simulink model "Example_for_the_implementation_of_the_inverse_kinematics"  (R2022a)
settings: Solver=FixedStepAuto  StartTime=0.0  StopTime=2  FixedStep=0.01  RelTol=1e-3  EnableMultiTasking=on
InitFcn:
  | %Simu_init
StopFcn:
  | %stop_sim
undefined symbols (not defined in the file): STIFF_FLOP_TipInverse
libraries: arduinolib x12, simulink x2, sldrtlib x1
settings Model: SimulationMode=external  PacingRate=1000  ExtModeTrigDuration=2  Creator=11010  LastModifiedBy=11010
settings SolverCC: AlgebraicLoopSolver=TrustRegion
settings OptimizationCC: EnhancedBackFolding=on  PassReuseOutputArgsAs=Individual arguments  MaxStackSize=64  OptimizeBlockOrder=speed  DifferentSizesBufferReuse=on  OptimizationCustomize=off  EfficientTunableParamExpr=on
settings DebuggingCC: ParameterTunabilityLossMsg=error  UnconnectedInputMsg=warning  UnconnectedOutputMsg=warning  UnconnectedLineMsg=warning  SFMachineParentedDataDiag=warning
settings HardwareCC: ProdBitPerPointer=32  ProdBitPerSizeT=32  ProdBitPerPtrDiffT=32  ProdLargestAtomicInteger=Long  ProdLargestAtomicFloat=Double  ProdWordSize=32  ProdHWDeviceType=ARM Compatible->ARM Cortex
settings SFSimCC: MATLABDynamicMemAlloc=off  CustomCodeUndefinedFunction=UseInterfaceOnly
settings RTWCC: SystemTargetFile=ert.tlc  HardwareBoard=Arduino Due  TemplateMakefile=ert_default_tmf  GenerateReport=on  Toolchain=Arduino ARM  BuildConfiguration=Faster Runs  IncludeHyperlinkInReport=on  LaunchReport=on  GenerateTraceInfo=on  GenerateTraceReport=on  GenerateTraceReportSl=on  GenerateTraceReportSf=on  GenerateTraceReportEml=on
settings CodeAppCC: ForceParamTrailComments=on  IgnoreCustomStorageClasses=off  OperatorAnnotations=on  SimulinkDataObjDesc=on  SFDataObjDesc=on  InsertBlockDesc=on
settings ERTTargetCC: SupportContinuousTime=on  SupportVariableSizeSignals=on  ExtModeTransport=3  ExtModeStaticAlloc=on  ExtModeStaticAllocSize=24576  ExtModeMexFile=ext_xcp  ExtModeIntrfLevel=Level2 - Open

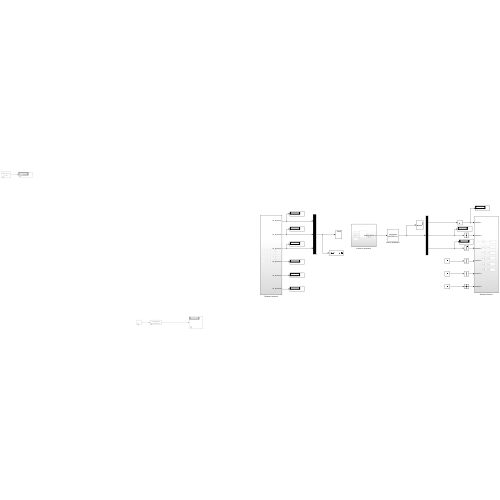
[thumbnail: Simulink's stored preview of the top-level diagram]
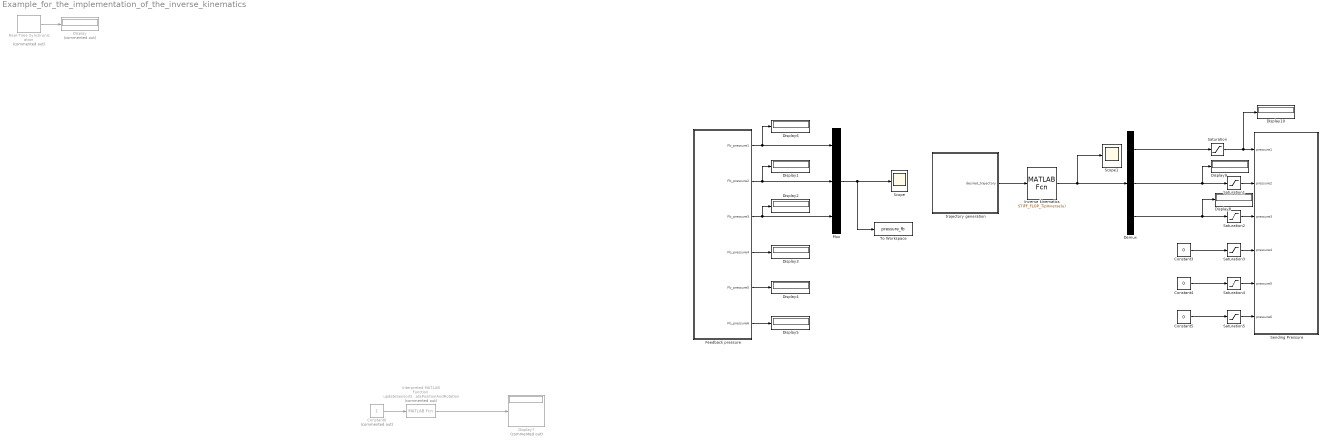
== system Example_for_the_implementation_of_the_inverse_kinematics ==
  Constant3 : Constant  Value=0
  Constant4 : Constant  Value=0
  Constant5 : Constant  Value=0
  Constant6 : Constant  Commented=on
  Demux : Demux  Outputs=3
  Display : Display  Commented=on
  Display{1..6,8..10} (9 alike) : Display
  Display7 : Display  Commented=on
  Feedback pressure : Subsystem
  Interpreted MATLAB Function : MATLABFcn  Commented=on  MATLABFcn=updateSensorDataPositionAndRotation  OutputDimensions=3
  Inverse kinematics : MATLABFcn  MATLABFcn=STIFF_FLOP_TipInverse(u)  OutputDimensions=3
  Mux : Mux  Inputs=3
  Real-Time Synchronization : sldrtlib/Real-Time Synchronization  Commented=on  SampleTime=0.1  MaxMissedTicks=100  ShowMissedTicks=on  YieldWhenWaiting=off
  Saturation{,1..5} (6 alike) : Saturate  UpperLimit=1.5  LowerLimit=0
  Scope : Scope
  Scope1 : Scope
  Sending Pressure : Subsystem
  To Workspace : ToWorkspace  VariableName=pressure_fb  SaveFormat=Structure With Time  SampleTime=-1
  trajectory generation : Subsystem
  wires:
  Demux/3 -> Saturation2/1, Display8/1
  Constant4/1 -> Saturation4/1
  Constant5/1 -> Saturation5/1
  Feedback pressure/2(Fb_pressure2) -> Display1/1, Mux/2
  Feedback pressure/3(Fb_pressure3) -> Display2/1, Mux/3
  Feedback pressure/4(Fb_pressure4) -> Display3/1
  Feedback pressure/5(Fb_pressure5) -> Display4/1
  Feedback pressure/6(Fb_pressure6) -> Display5/1
  Feedback pressure/1(Fb_pressure1) -> Display6/1, Mux/1
  Real-Time Synchronization/1 -> Display/1
  Constant3/1 -> Saturation3/1
  Interpreted MATLAB Function/1 -> Display7/1
  Constant6/1 -> Interpreted MATLAB Function/1
  Saturation/1 -> Display10/1, Sending Pressure/1(pressure1)
  Saturation1/1 -> Sending Pressure/2(pressure2)
  Saturation2/1 -> Sending Pressure/3(pressure3)
  Saturation3/1 -> Sending Pressure/4(pressure4)
  Saturation4/1 -> Sending Pressure/5(pressure5)
  Saturation5/1 -> Sending Pressure/6(pressure6)
  Inverse kinematics/1 -> Scope1/1, Demux/1
  trajectory generation/1(desired_trajectory) -> Inverse kinematics/1
  Mux/1 -> To Workspace/1, Scope/1
  Demux/1 -> Saturation/1
  Demux/2 -> Display9/1, Saturation1/1

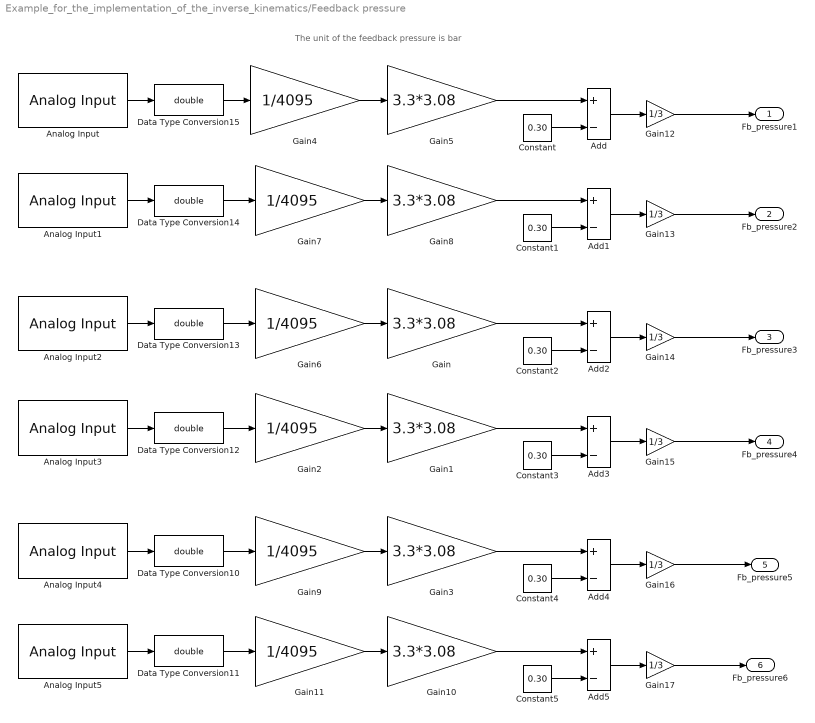
== system Example_for_the_implementation_of_the_inverse_kinematics/Feedback pressure ==
  note: The unit of the feedback pressure is bar
  Add{,1..5} (6 alike) : Sum  Inputs=+-
  Analog Input : arduinolib/Analog Input  pinNumber=0  ReadResultsOnly=off  ConversionTriggerSource=Software  ExternalTriggerType=uint32(0)  OutputDataType=uint16  EnableConversionCompleteNotify=off  EnableOuputStatus=off  SampleTime=0.01  blockPlatform=arduino
  Analog Input1 : arduinolib/Analog Input  pinNumber=1  ReadResultsOnly=off  ConversionTriggerSource=Software  ExternalTriggerType=uint32(0)  OutputDataType=uint16  EnableConversionCompleteNotify=off  EnableOuputStatus=off  SampleTime=0.01  blockPlatform=arduino
  Analog Input2 : arduinolib/Analog Input  pinNumber=2  ReadResultsOnly=off  ConversionTriggerSource=Software  ExternalTriggerType=uint32(0)  OutputDataType=uint16  EnableConversionCompleteNotify=off  EnableOuputStatus=off  SampleTime=0.01  blockPlatform=arduino
  Analog Input3 : arduinolib/Analog Input  pinNumber=3  ReadResultsOnly=off  ConversionTriggerSource=Software  ExternalTriggerType=uint32(0)  OutputDataType=uint16  EnableConversionCompleteNotify=off  EnableOuputStatus=off  SampleTime=0.01  blockPlatform=arduino
  Analog Input4 : arduinolib/Analog Input  pinNumber=4  ReadResultsOnly=off  ConversionTriggerSource=Software  ExternalTriggerType=uint32(0)  OutputDataType=uint16  EnableConversionCompleteNotify=off  EnableOuputStatus=off  SampleTime=0.01  blockPlatform=arduino
  Analog Input5 : arduinolib/Analog Input  pinNumber=5  ReadResultsOnly=off  ConversionTriggerSource=Software  ExternalTriggerType=uint32(0)  OutputDataType=uint16  EnableConversionCompleteNotify=off  EnableOuputStatus=off  SampleTime=0.01  blockPlatform=arduino
  Constant{,1..5} (6 alike) : Constant  Value=0.30
  Data Type Conversion{10..15} (6 alike) : DataTypeConversion  OutDataTypeStr=double  SaturateOnIntegerOverflow=off  RndMeth=Floor
  Gain{,1,3,5,8,10} (6 alike) : Gain  Gain=3.3*3.08
  Gain{2,4,6..7,9,11} (6 alike) : Gain  Gain=1/4095
  Gain{12..17} (6 alike) : Gain  Gain=1/3
  Fb_pressure1 : Outport
  Fb_pressure2 : Outport  Port=2
  Fb_pressure3 : Outport  Port=3
  Fb_pressure4 : Outport  Port=4
  Fb_pressure5 : Outport  Port=5
  Fb_pressure6 : Outport  Port=6
  wires:
  Analog Input2/1 -> Data Type Conversion13/1
  Analog Input1/1 -> Data Type Conversion14/1
  Analog Input/1 -> Data Type Conversion15/1
  Analog Input5/1 -> Data Type Conversion11/1
  Analog Input3/1 -> Data Type Conversion12/1
  Analog Input4/1 -> Data Type Conversion10/1
  Gain5/1 -> Add/1
  Add/1 -> Gain12/1
  Gain13/1 -> Fb_pressure2/1
  Data Type Conversion13/1 -> Gain6/1
  Data Type Conversion15/1 -> Gain4/1
  Data Type Conversion12/1 -> Gain2/1
  Data Type Conversion10/1 -> Gain9/1
  Gain6/1 -> Gain/1
  Gain4/1 -> Gain5/1
  Data Type Conversion14/1 -> Gain7/1
  Gain7/1 -> Gain8/1
  Gain2/1 -> Gain1/1
  Gain9/1 -> Gain3/1
  Data Type Conversion11/1 -> Gain11/1
  Gain11/1 -> Gain10/1
  Constant/1 -> Add/2
  Gain12/1 -> Fb_pressure1/1
  Gain8/1 -> Add1/1
  Constant1/1 -> Add1/2
  Add1/1 -> Gain13/1
  Add2/1 -> Gain14/1
  Constant2/1 -> Add2/2
  Gain/1 -> Add2/1
  Gain14/1 -> Fb_pressure3/1
  Add3/1 -> Gain15/1
  Constant3/1 -> Add3/2
  Gain1/1 -> Add3/1
  Gain15/1 -> Fb_pressure4/1
  Gain16/1 -> Fb_pressure5/1
  Gain3/1 -> Add4/1
  Add4/1 -> Gain16/1
  Constant4/1 -> Add4/2
  Gain10/1 -> Add5/1
  Gain17/1 -> Fb_pressure6/1
  Add5/1 -> Gain17/1
  Constant5/1 -> Add5/2

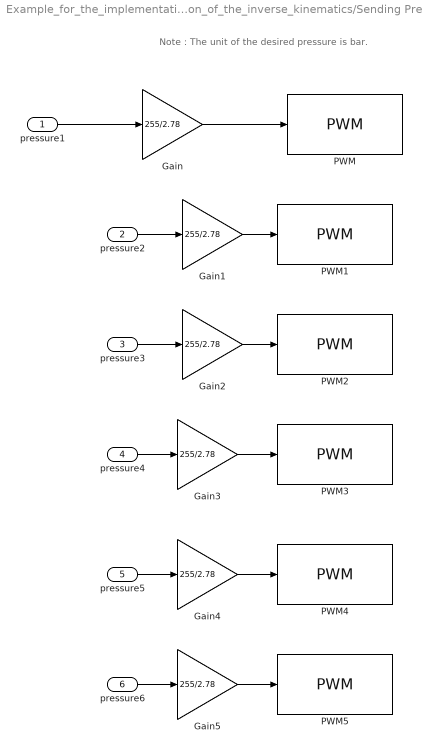
== system Example_for_the_implementation_of_the_inverse_kinematics/Sending Pressure ==
  note: Note : The unit of the desired pressure is bar.
  pressure1 : Inport
  pressure2 : Inport  Port=2
  pressure3 : Inport  Port=3
  pressure4 : Inport  Port=4
  pressure5 : Inport  Port=5
  pressure6 : Inport  Port=6
  Gain{,1..5} (6 alike) : Gain  Gain=255/2.78
  PWM : arduinolib/PWM  pinNumber=2  frequencyType=Default  desiredFrequency=490.2  achievableFrequency=490.2
  PWM1 : arduinolib/PWM  pinNumber=3  frequencyType=Default  desiredFrequency=490.2  achievableFrequency=490.2
  PWM2 : arduinolib/PWM  pinNumber=5  frequencyType=Default  desiredFrequency=490.2  achievableFrequency=490.2
  PWM3 : arduinolib/PWM  pinNumber=6  frequencyType=Default  desiredFrequency=490.2  achievableFrequency=490.2
  PWM4 : arduinolib/PWM  pinNumber=7  frequencyType=Default  desiredFrequency=490.2  achievableFrequency=490.2
  PWM5 : arduinolib/PWM  pinNumber=8  frequencyType=Default  desiredFrequency=490.2  achievableFrequency=490.2
  wires:
  pressure6/1 -> Gain5/1
  pressure3/1 -> Gain2/1
  pressure5/1 -> Gain4/1
  pressure4/1 -> Gain3/1
  pressure2/1 -> Gain1/1
  Gain/1 -> PWM/1
  Gain1/1 -> PWM1/1
  Gain2/1 -> PWM2/1
  Gain3/1 -> PWM3/1
  Gain4/1 -> PWM4/1
  Gain5/1 -> PWM5/1
  pressure1/1 -> Gain/1

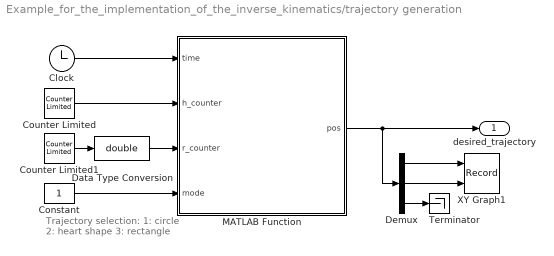
== system Example_for_the_implementation_of_the_inverse_kinematics/trajectory generation ==
  note: Trajectory selection:
      | 1: circle
      | 2: heart shape
      | 3: rectangle
  Clock : Clock
  Constant : Constant
  Counter Limited : simulink/Sources/Counter Limited  uplimit=89  tsamp=-1
  Counter Limited1 : simulink/Sources/Counter Limited  uplimit=79  tsamp=-1
  Data Type Conversion : DataTypeConversion  OutDataTypeStr=double  SaturateOnIntegerOverflow=off  RndMeth=Floor
  Demux : Demux  Outputs=3
  MATLAB Function : MATLAB Function  TreatAsAtomicUnit=on
  Terminator : Terminator
  XY Graph1 : Record  FileSettingsInternal="{\"entries\":[{\"content\":{\"excelSettings\":{\"content\":{},\"type\":\"Streamout.ExcelSettings\"}},\"type\":\"Streamout.FileSettingStorage\",\"uuid\":\"82168634-0a0a-45a7-af1b-8dfb82ff34b5\"}],\"packageUris\":[\"http://schema.mathworks.com/mf0/streamout_blocks/R2020a\"],\"version\":\"1.0\"}"  Layout=[1 1]  SignalsInternal="{\"entries\":[{\"content\":{\"signals\":[{\"content\":{\"blockPath\":[\"Example_for_the_implementation_of_the_inverse_kinematics/trajectory generation/XY Graph1\"],\"channel\":[],\"dimensions\":[1,1],\"domain\":\"Example_for_the_implementation_of_the_inverse_kinematics/trajectory generation/XY Graph1\",\"lineColor\":\"#a2142f\",\"plots\":[1],\"port\":1,\"sid\":[],\"signalID\":9,\"signalName\":\"Demux:1\"},\"type\":\"RecordBlkView.Signal\",\"uuid\":\"e88520da-0b60-493b-89f6-a2fcb696c124\"},{\"content\":{\"blockPath\":[\"Example_for_the_implementation_of_the_inverse_kinematics/trajectory generation/XY Graph1\"],\"channel\":[],\"dimensions\":[1,1],\"domain\":\"Example_for_the_implementation_of_the_inverse_kinematics/trajectory generation/XY Graph1\",\"lineColor\":\"#139fff\",\"plots\":[1],\"port\":2,\"sid\":[],\"signalID\":12,\"signalName\":\"Demux:2\"},\"type\":\"RecordBlkView.Signal\",\"uuid\":\"3da2b6d2-c75c-45d3-af78-59041fc211a0\"}]},\"type\":\"RecordBlkView.InputSignals\",\"uuid\":\"50cdf598-2aac-4fcc-8ebd-bf93376f4c44\"}],\"packageUris\":[\"http://schema.mathworks.com/mf0/streamout_blocks/R2020a\"],\"version\":\"1.0\"}"  VisualizationBindings="{\"xyplotplugin\":{\"info\":[{\"series\":[{\"bindingParametersList\":[{\"parameter\":\"X-Axis\",\"signalID\":9,\"signalName\":\"Demux:1\"},{\"parameter\":\"Y-Axis\",\"signalID\":12,\"signalName\":\"Demux:2\"}],\"seriesID\":10653}],\"subplotID\":1}]}}"  CompatibilityTag=XY  st=-1
  desired_trajectory : Outport
  wires:
  MATLAB Function/1(pos) -> desired_trajectory/1, Demux/1
  Demux/2 -> XY Graph1/2
  Demux/1 -> XY Graph1/1
  Demux/3 -> Terminator/1
  Counter Limited1/1 -> Data Type Conversion/1
  Constant/1 -> MATLAB Function/4(mode)
  Data Type Conversion/1 -> MATLAB Function/3(r_counter)
  Counter Limited/1 -> MATLAB Function/2(h_counter)
  Clock/1 -> MATLAB Function/1(time)

== matlab function Example_for_the_implementation_of_the_inverse_kinematics/trajectory generation/MATLAB Function ==
  data: time input; h_counter input; r_counter input; pos output; mode input
function pos = trajectory_generation(time,h_counter,r_counter, mode)
pos_z = 0.05;
    if mode == 1
        % define the rotation speed
        omega = 2*pi;
        % define the radius
        r = 0.015;
        % trajectory generation
        pos = [r*cos(omega*time); r*sin(omega*time); pos_z];
    elseif mode == 2
        r = 0.04;
        space = linspace(-pi,pi,90);
        space_point = space(h_counter + 1);
        x = 0.18*r*space_point*sin(pi*0.872*sin(space_point)/space_point);
        y = -r*0.18*abs(space_point)*cos(pi*sin(space_point)/space_point);
        pos = [x;y;pos_z];
    else
        if r_counter <= 10
            x = 0.015;
            y = 0.0015*(r_counter);
        elseif r_counter <= 30
            y = 0.015;
            x = 0.015 - 0.0015*(r_counter-10);
        elseif r_counter <= 50
            x = -0.015;
            y = 0.015 - 0.0015*(r_counter-30);
        elseif r_counter <= 70
            y = -0.015;
            x = -0.015 + 0.0015*(r_counter-50);
        else
            x = 0.015;
            y = -0.015+0.0015*(r_counter-70);
        end
        pos = [x;y;pos_z];
    end
